simulink model "Model_I6_Rigid_Pitch"  (Simulink 6.6)
settings: Solver=ode45  StartTime=tmin  StopTime=tmax  MaxStep=dt  RelTol=1e-3
values from neighbouring files (symbols this model uses):
  dt = 0.01    [Pgm_G11_Superposition.m]    (also in Pgm_G12_Num_Integration.m; Pgm_G13_Frequency_Domain.m = 0.0625; Pgm_H2_Response_Gusts_Control.m = 0.001; Pgm_H3_Ase_Gusts_Pid.m = 0.001)
  MC = inv(A)*C    [Pgm_H2_Response_Gusts_Control.m]    (also in Pgm_H3_Ase_Gusts_Pid.m; Pgm_I6_Dynamic_Manoeuvres.m = inv(M) * C; Pgm_I7_Gust_Time.m = MI * CC; Pgm_I91_Taxiing.m = inv(M) * CC)
  MF = inv(M) * F    [Pgm_I6_Dynamic_Manoeuvres.m]
settings Model: Creator=Jan Wright  LastModifiedBy=Jan Wright
settings DataIOCC: SignalLoggingName=sigsOut
settings DebuggingCC: SignalResolutionControl=TryResolveAllWithWarning  SolverPrmCheckMsg=none  MultiTaskDSMMsg=warning  MultiTaskCondExecSysMsg=none  StrictBusMsg=None
settings HardwareCC: TargetUnknown=on
settings RTWCC: IncludeERTFirstTime=on
settings GRTTargetCC: ModelReferenceCompliant=off  MatFileLogging=off

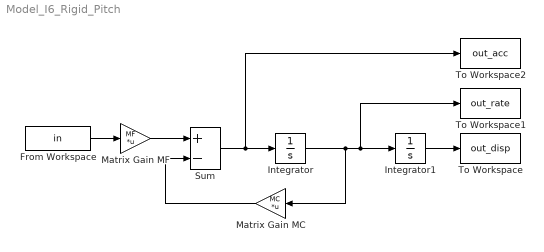
== system Model_I6_Rigid_Pitch ==
  From Workspace : FromWorkspace  VariableName=in  SampleTime=dt
  Integrator : Integrator
  Integrator1 : Integrator
  Matrix Gain MC : Gain  Orientation=left  Gain=MC  Multiplication=Matrix(K*u)  SampleTime=dt  SaturateOnIntegerOverflow=on
  Matrix Gain MF : Gain  Gain=MF  Multiplication=Matrix(K*u)  SampleTime=dt  SaturateOnIntegerOverflow=on
  Sum : Sum  Inputs=+-  SaturateOnIntegerOverflow=on
  To Workspace : ToWorkspace  VariableName=out_disp  SampleTime=dt  SaveFormat=Array
  To Workspace1 : ToWorkspace  VariableName=out_rate  SampleTime=dt  SaveFormat=Array
  To Workspace2 : ToWorkspace  VariableName=out_acc  SampleTime=dt  SaveFormat=Array
  wires:
  From Workspace/1 -> Matrix Gain MF/1
  Matrix Gain MF/1 -> Sum/1
  Sum/1 -> Integrator/1, To Workspace2/1
  Integrator/1 -> Matrix Gain MC/1, Integrator1/1, To Workspace1/1
  Matrix Gain MC/1 -> Sum/2
  Integrator1/1 -> To Workspace/1
